simulink model "untitled11"  (R2017b)
settings: Solver=FixedStepAuto  StartTime=0.0  StopTime=10.0  FixedStep=0.00001  RelTol=1e-3
undefined symbols (not defined in the file or in its folder): magnitude
libraries: simulink x1
settings Model: Creator=user  LastModifiedBy=user

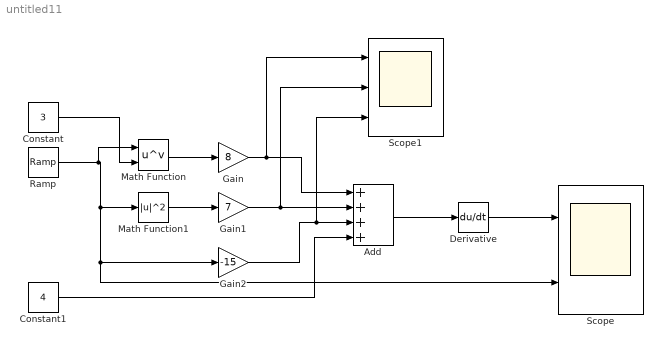
== system untitled11 ==
  Add : Sum  Inputs=4
  Constant : Constant  Value=3
  Constant1 : Constant  Value=4
  Derivative : Derivative  CoefficientInTFapproximation=1
  Gain : Gain  Gain=8
  Gain1 : Gain  Gain=7
  Gain2 : Gain  Gain=-15
  Math Function : Math  Operator=pow  OutputSignalType=real  SaturateOnIntegerOverflow=on
  Math Function1 : Math  Operator=magnitude^2  OutputSignalType=real  SaturateOnIntegerOverflow=on
  Ramp : simulink/Sources/Ramp  slope=1  start=0  X0=0
  Scope : Scope  NumInputPorts=2
  Scope1 : Scope  NumInputPorts=3
  wires:
  Ramp/1 -> Math Function/1, Scope/2, Gain2/1, Math Function1/1
  Math Function/1 -> Gain/1
  Math Function1/1 -> Gain1/1
  Gain/1 -> Scope1/1, Add/1
  Gain1/1 -> Scope1/2, Add/2
  Gain2/1 -> Scope1/3, Add/3
  Constant1/1 -> Add/4
  Add/1 -> Derivative/1
  Derivative/1 -> Scope/1
  Constant/1 -> Math Function/2
